simulink model "PositionControlSystem"  (R2018a)
settings: Solver=VariableStepAuto  StartTime=0.0  StopTime=5  RelTol=1e-3
libraries: simulink x1
settings Model: Creator=Deano  LastModifiedBy=Deano
settings OptimizationCC: DefaultParameterBehavior=Inlined  UseDivisionForNetSlopeComputation=on  UseFloatMulNetSlope=on  InlineInvariantSignals=on  PassReuseOutputArgsAs=Individual arguments  ZeroExternalMemoryAtStartup=off  ZeroInternalMemoryAtStartup=off  NoFixptDivByZeroProtection=on  EfficientFloat2IntCast=on  LifeSpan=1  OptimizeBlockOrder=speed  DifferentSizesBufferReuse=on
settings DebuggingCC: ParameterTunabilityLossMsg=error
settings HardwareCC: ProdLongLongMode=on
settings SFSimCC: MATLABDynamicMemAlloc=off
settings RTWCC: SystemTargetFile=ert.tlc  TemplateMakefile=ert_default_tmf  GenerateReport=on  IncludeHyperlinkInReport=on  LaunchReport=on  TargetLang=C++  GenerateTraceInfo=on  GenerateTraceReport=on  GenerateTraceReportSl=on  GenerateTraceReportSf=on  GenerateTraceReportEml=on
settings CodeAppCC: ForceParamTrailComments=on  IgnoreCustomStorageClasses=off  OperatorAnnotations=on  SimulinkDataObjDesc=on  SFDataObjDesc=on  CustomSymbolStrGlobalVar=rt$N$M  CustomSymbolStrType=$N$M  CustomSymbolStrFcn=$N$M$F  CustomSymbolStrMacro=$N$M  InsertBlockDesc=on
settings ERTTargetCC: TargetLangStandard=C++03 (ISO)  GenerateSampleERTMain=on  IncludeMdlTerminateFcn=off  CombineSignalStateStructs=on  MultiInstanceERTCode=on  CodeInterfacePackaging=C++ class  SupportComplex=off  SupportContinuousTime=on  InlinedParameterPlacement=NonHierarchical  RootIOFormat=Structure reference  ERTCustomFileTemplate=example_file_process.tlc  ERTFilePackagingFormat=CompactWithDataFile

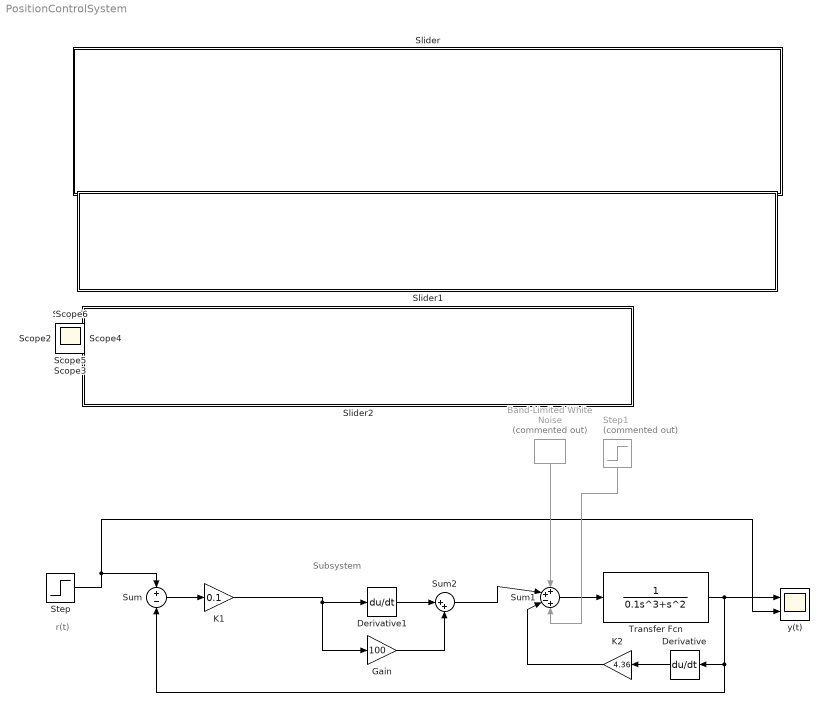
== system PositionControlSystem ==
  note: Subsystem
  note: r(t)
  Band-Limited White Noise : simulink/Sources/Band-Limited White Noise  Commented=on  Cov=.1  Ts=0.01  seed=[23341]
  Derivative : Derivative  CoefficientInTFapproximation=0
  Derivative1 : Derivative  CoefficientInTFapproximation=0
  Gain : Gain  Gain=100
  K1 : Gain  Gain=0.1
  K2 : Gain  Gain=4.36
  Slider : Subsystem  DialogController=hmiCreateDDGDialog  IsWebBlock=on  mask(MWDashboardBlock){webBlockId=00ac4b92-4e85-4a9c-87f5-90d0529770bf, webBlockType=slider, ShowInLibBrowser=on, ShowInitialText=on, HMISrcModelName=PositionControlSystem}
      mask prompts: webBlockId "WebBlock Id"; webBlockType "WebBlock Type"; HMISrcModelName "Source Model"
      mask help: SimulinkHMI:dialogs:SliderDialogDesc
      mask Help: helpview([docroot '/mapfiles/simulink.map'], 'hmi_slider')
      mask Display:
      | if strcmp(get_param(bdroot(gcb),'BlockDiagramType'), 'library')
      |     image([(matlabroot) '/toolbox/simulink/hmi/icons/Slider.png']);
      | end
  Slider1 : Subsystem  DialogController=hmiCreateDDGDialog  IsWebBlock=on  mask(MWDashboardBlock){webBlockId=da2f7c1d-5a0f-4431-b4c9-2f0478c40cc5, webBlockType=slider, ShowInLibBrowser=on, ShowInitialText=on, HMISrcModelName=PositionControlSystem}
      mask prompts: webBlockId "WebBlock Id"; webBlockType "WebBlock Type"; HMISrcModelName "Source Model"
      mask help: SimulinkHMI:dialogs:SliderDialogDesc
      mask Help: helpview([docroot '/mapfiles/simulink.map'], 'hmi_slider')
      mask Display:
      | if strcmp(get_param(bdroot(gcb),'BlockDiagramType'), 'library')
      |     image([(matlabroot) '/toolbox/simulink/hmi/icons/Slider.png']);
      | end
  Slider2 : Subsystem  DialogController=hmiCreateDDGDialog  IsWebBlock=on  mask(MWDashboardBlock){webBlockId=7d2787ed-fee8-476d-8e28-a3caa0679abc, webBlockType=slider, ShowInLibBrowser=on, ShowInitialText=on, HMISrcModelName=PositionControlSystem}
      mask prompts: webBlockId "WebBlock Id"; webBlockType "WebBlock Type"; HMISrcModelName "Source Model"
      mask help: SimulinkHMI:dialogs:SliderDialogDesc
      mask Help: helpview([docroot '/mapfiles/simulink.map'], 'hmi_slider')
      mask Display:
      | if strcmp(get_param(bdroot(gcb),'BlockDiagramType'), 'library')
      |     image([(matlabroot) '/toolbox/simulink/hmi/icons/Slider.png']);
      | end
  Step : Step  SampleTime=0.001
  Step1 : Step  Commented=on  SampleTime=0
  Sum : Sum  Inputs=+-
  Sum1 : Sum  Inputs=++-+
  Sum2 : Sum  Inputs=|++
  Transfer Fcn : TransferFcn  Denominator=[0.1 1 0 0]  AbsoluteTolerance=1e10
  y(t) : Scope  NumInputPorts=2
  Scope{,1..6} (7 alike) : Scope
  wires:
  Sum1/1 -> Transfer Fcn/1
  Sum/1 -> K1/1
  Step/1 -> y(t)/2, Sum/1
  Transfer Fcn/1 -> Sum/2, Derivative/1, y(t)/1
  Derivative/1 -> K2/1
  Derivative1/1 -> Sum2/1
  Gain/1 -> Sum2/2
  Sum2/1 -> Sum1/2
  Band-Limited White Noise/1 -> Sum1/1
  K1/1 -> Gain/1, Derivative1/1
  K2/1 -> Sum1/3
  Step1/1 -> Sum1/4

== system PositionControlSystem/Slider ==

== system PositionControlSystem/Slider1 ==

== system PositionControlSystem/Slider2 ==
